simulink model "untitled"  (R2023b)
settings: Solver=VariableStepAuto  StartTime=0.0  StopTime=10.0  RelTol=1e-3
undefined symbols (not defined in the file): factstruct
libraries: aerolibatmos2 x1, aerolibadyn x1, aerolibwind2 x1
settings Model: Creator=kaleb  LastModifiedBy=kaleb

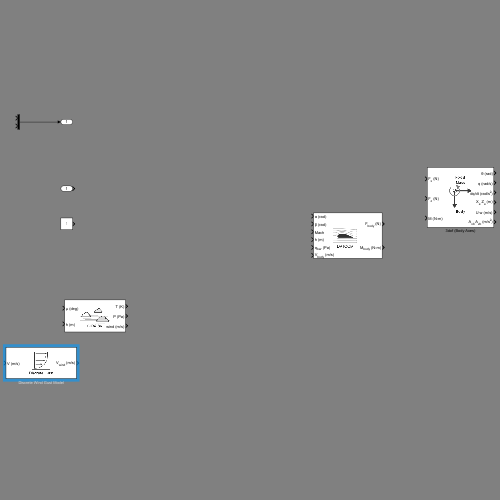
[thumbnail: Simulink's stored preview of the top-level diagram]
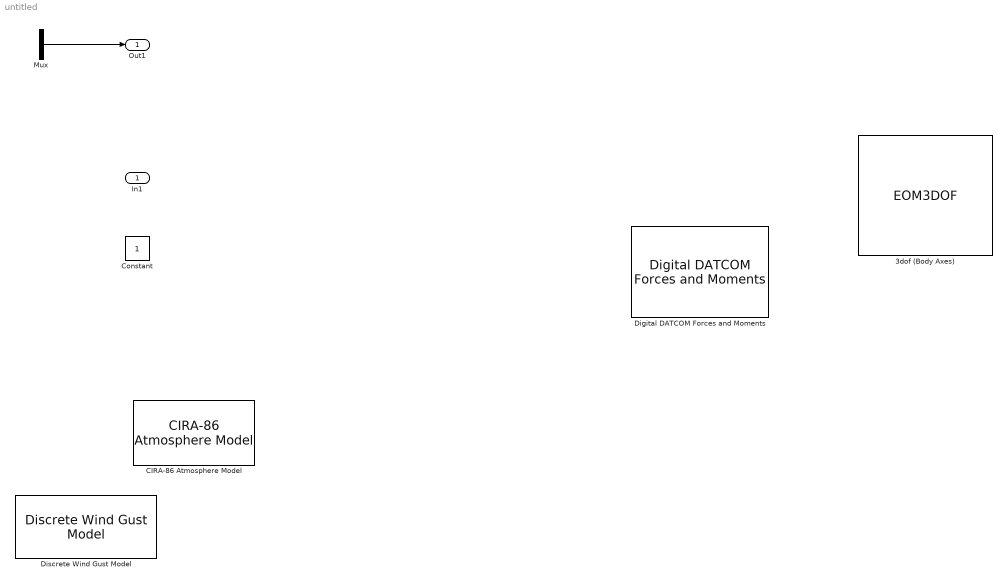
== system untitled ==
  In1 : Inport
  3dof (Body Axes) : EOM3DOF
  CIRA-86 Atmosphere Model : aerolibatmos2/CIRA-86 Atmosphere Model  units=Metric (MKS)  ctype=GPHeight  mtype=Monthly  month=January  action=Warning
  Constant : Constant
  Digital DATCOM Forces and Moments : aerolibadyn/Digital DATCOM Forces and Moments  units=Metric (MKS)  dcase=factstruct{1}  fmode=Body  buildno=0  imethod=Linear  emethod=None - clip  rmethod=Clip to Range  action=Warning
  Discrete Wind Gust Model : aerolibwind2/Discrete Wind Gust Model  units=Metric (MKS)  Gx=on  Gy=on  Gz=on  t_0=5  d_m=[120 120 80]  v_m=[3.5 3.5 3.0]
  Mux : Mux  Inputs=2
  Out1 : Outport
  wires:
  Mux/1 -> Out1/1
